simulink model "Att_Ctrl"  (Simulink 8.0)
settings: configuration reference "configSetObj_autopilot" (kept outside this file)
undefined symbols (not defined in the file or in its folder): cmdLim, dispGain, dispLim, intGain, rateGain, rateLim
undefined symbols (not defined in the file): intLim
libraries: simulink x1
settings Model: RequirementInfo={} %GIDa_eb906a4c_0ec7_43a1_b5c3_86a9990349a4  reqMgrSettings="100 S'doors','misc'{{S'surrogatepath','savemodel','savesurrogate','doorsLinks2sl','slLinks2Doors','detaillevel','surrogateId','synctime'{{T\"/Autopilot Project/attitude_controller\",M[1],M[1],M[1],M[1],M[1],T\"00000040\",T\"\"}},S'mode','pathStorage'{{T\"generic\",T\"modelRelative\"}}}}"  Creator=bpotter  LastModifiedBy=ssauvage  RecordCoverage=on  CovSaveName=attitude_controller_covdata  CovMetricSettings=dcmtrwe  CovHTMLOptions=-aTS=1 -bRG=1 -bTC=1 -hTR=1 -nFC=0 -scm=1 -bcm=1  CovHtmlReporting=off  CovCumulativeVarName=attitude_controller_covCumulativeData  CovCumulativeReport=on  CovReportOnPause=off
settings ConfigSet: SourceLocation=Base Workspace

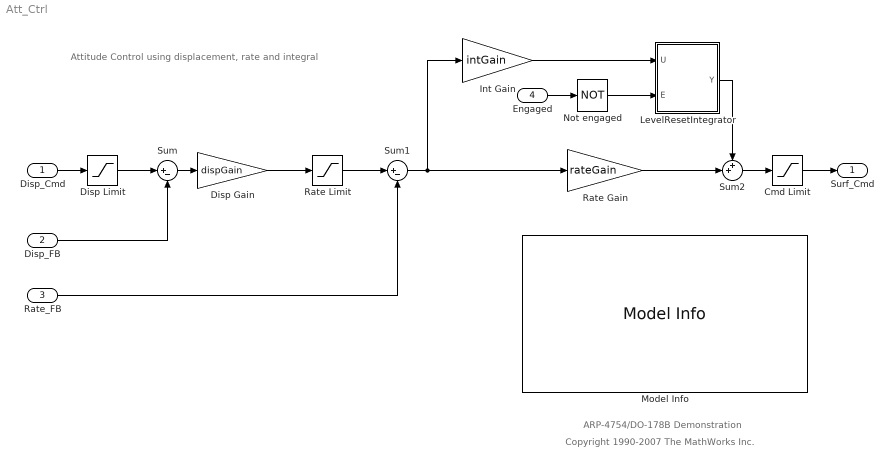
== system Att_Ctrl ==
  note: Attitude Control using displacement, rate and integral
  note: Copyright 1990-2007 The MathWorks Inc.
  note: ARP-4754/DO-178B Demonstration
  Disp_Cmd : Inport  RequirementInfo={} %GIDa_1f6c7271_93c3_4f3b_ad46_40b2620097e5  OutDataTypeStr=double  PortDimensions=1  SampleTime=1/40
  "Disp_FB " : Inport  RequirementInfo={} %GIDa_a4c10b54_79b2_494f_9fbb_11aba459525d  Port=2  OutDataTypeStr=double  PortDimensions=1  SampleTime=1/40
  Rate_FB : Inport  RequirementInfo={} %GIDa_8a5ee350_5b96_4034_aa7b_307fc7a5da71  Port=3  OutDataTypeStr=double  PortDimensions=1  SampleTime=1/40
  Engaged : Inport  RequirementInfo={} %GIDa_99509e30_ac8c_4d41_82c3_48695d972b31  Port=4  OutDataTypeStr=boolean  PortDimensions=1  SampleTime=1/40
  Cmd Limit : Saturate  RequirementInfo={} %GIDa_ec5fb8d1_63e1_4cbf_bd50_e97ea1f3a86f  UpperLimit=cmdLim  LowerLimit=-cmdLim
      settings: AttributesFormatString=%<LowerLimit> to %<UpperLimit> (deg)
  Disp Gain : Gain  RequirementInfo={} %GIDa_4fcfcfe9_3275_4fa9_885f_cf306a71b936  Gain=dispGain
  Disp Limit : Saturate  RequirementInfo={} %GIDa_7b92da27_c5ec_485b_a9fa_f73a890a94ea  UpperLimit=dispLim  LowerLimit=-dispLim
      settings: AttributesFormatString=%<LowerLimit> to %<UpperLimit> (deg)
  Int Gain : Gain  RequirementInfo={} %GIDa_beea6fba_2894_42ca_8163_07bc86b02f8e  Gain=intGain
  LevelResetIntegrator : Subsystem  RequirementInfo={} %GIDa_62f927bb_12b1_4b21_a854_7eb9263471c0  mask(SLCI_Level_Reset_Integrator){K=1.0, Ts=1/40, IC=0, UL=intLim, LL=-intLim}
      mask prompts: K "Gain value:"; Ts "Sample time (-1 for inherited):"; IC "Initial condition:"; UL "Upper saturation limit:"; LL "Lower saturation limit:"
      mask help: Level reset integrator using Forward Euler method. This masked subsystem implements the functional behavior of Simulink's Descrete-Time Integrator block using Simulink Code Inspector supported blocks.
      settings: AttributesFormatString=-%<LL> to %<UL>\n(deg)
      mask Display: fprintf('K Ts\n____\nz-1')
  Model Info : simulink/Model-Wide Utilities/Model Info  RequirementInfo={} %GIDa_c5788dca_0805_4822_8543_5a51a7c0beb7  InitialBlockCM=None  BlockCM=None  Frame=on  DisplayStringWithTags=|  HorizontalTextAlignment=Left  LeftAlignmentValue=0.02  SourceBlockDiagram=Att_Ctrl  TagMaxNumber=20
      | Attitude Controller
      | Author: %<LastModifiedBy>
      | Version: %<ModelVersion>
      | Date: %<LastModificationDate>
      | DO-178B Software Lifecycle Data:
      |   11.9 Software Requirements Data
      |   11.10 Design Description
      | DO-178B Objectives:
      |   5.2.1a Low Level Requirements are Developed
      |   5.2.1a Software Architecture is Developed
      |   5.2.1b  Derived Low Level Requirements are Developed
  Not engaged : Logic  RequirementInfo={} %GIDa_955db51c_db14_42aa_b67d_de05482530f8  Operator=NOT  IconShape=distinctive  AllPortsSameDT=off  OutDataTypeStr=boolean
  Rate Gain : Gain  RequirementInfo={} %GIDa_4fe20f02_adbd_4ca0_a7f6_fed161d48486  Gain=rateGain
  Rate Limit : Saturate  RequirementInfo={} %GIDa_6ae337a4_f989_4d2e_9517_e05a98139e9b  UpperLimit=rateLim  LowerLimit=-rateLim
      settings: AttributesFormatString=%<LowerLimit> to %<UpperLimit> (deg/sec)
  Sum : Sum  RequirementInfo={} %GIDa_cf5e480a_5b22_4e1a_9467_aeba7515f114  Inputs=|+-
  Sum1 : Sum  RequirementInfo={} %GIDa_37a43aee_ff03_4021_a10a_39656d6638a3  Inputs=|+-
  Sum2 : Sum  RequirementInfo={} %GIDa_fadb0a26_a1fd_480b_9f5d_0b7f45001c5e  Inputs=++|
  Surf_Cmd : Outport  RequirementInfo={} %GIDa_99d2b8ce_ab27_4685_9887_a082a0698432  OutDataTypeStr=double  PortDimensions=1  SampleTime=1/40
  wires:
  Disp_Cmd/1 -> Disp Limit/1
  "Disp_FB "/1 -> Sum/2
  Rate_FB/1 -> Sum1/2
  Sum1/1 -> Rate Gain/1, Int Gain/1
  Disp Gain/1 -> Rate Limit/1
  Sum/1 -> Disp Gain/1
  Disp Limit/1 -> Sum/1
  Rate Limit/1 -> Sum1/1
  Cmd Limit/1 -> Surf_Cmd/1
  Rate Gain/1 -> Sum2/2
  Sum2/1 -> Cmd Limit/1
  Engaged/1 -> Not engaged/1
  Not engaged/1 -> LevelResetIntegrator/2(E)
  LevelResetIntegrator/1(Y) -> Sum2/1
  Int Gain/1 -> LevelResetIntegrator/1(U)

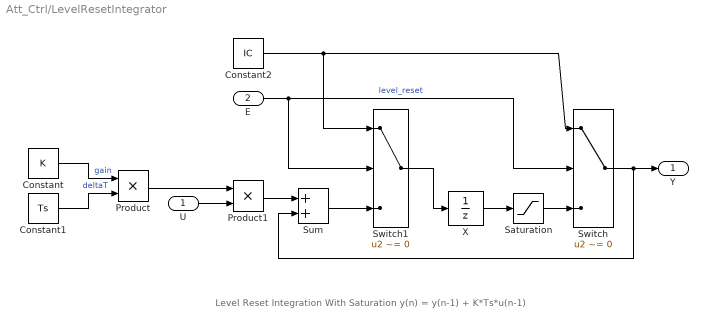
== system Att_Ctrl/LevelResetIntegrator ==
  note: Level Reset Integration With Saturation
      | y(n) = y(n-1) + K*Ts*u(n-1)
  U : Inport
  E : Inport  Port=2
  Constant : Constant  Value=K
  Constant1 : Constant  Value=Ts
  Constant2 : Constant  Value=IC
  Product : Product  RndMeth=Zero
  Product1 : Product  RndMeth=Zero
  Saturation : Saturate  UpperLimit=UL  LowerLimit=LL
  Sum : Sum
  Switch : Switch  Criteria=u2 ~= 0
  Switch1 : Switch  Criteria=u2 ~= 0
  X : UnitDelay  InitialCondition=IC  SampleTime=Ts
  Y : Outport
  wires:
  Switch/1 -> Sum/2, Y/1
  Constant2/1 -> Switch/1, Switch1/1
  Saturation/1 -> Switch/3
  Product1/1 -> Sum/1
  X/1 -> Saturation/1
  U/1 -> Product1/2
  Product/1 -> Product1/1
  Constant1/1 -> Product/2  "deltaT"
  Constant/1 -> Product/1  "gain"
  Switch1/1 -> X/1
  Sum/1 -> Switch1/3
  E/1 -> Switch/2, Switch1/2  "level_reset"
